simulink model "Missile_Trim_Verification"  (R2021b)
settings: Solver=ode4  StartTime=0.0  StopTime=20  FixedStep=Step_Size  RelTol=1e-3
InitFcn:
  | Missile_Data;
  | Sim_Parameters;
values from neighbouring files (symbols this model uses):
  Init_Euler = x_trim(7:9)    [Sim_Parameters.m]
  Init_Rate = x_trim(4:6)    [Sim_Parameters.m]
  Init_Vel = x_trim(1:3)    [Sim_Parameters.m]
  UNIT_GRAV = 9.81    [Sim_Parameters.m]
undefined symbols (not defined in the file or in its folder): CTC, D, G_turn, gamma_trim, h_trim, Mass, psi_dot_trim, ROC, S, SC, Tbl_CL_ALPHAT, Tbl_CL_DEL_R, Tbl_CL_P, Tbl_CM_0, Tbl_CM_DEL_P, Tbl_CM_PHIT, Tbl_CM_Q, Tbl_CN_DEL_Y, Tbl_CN_PHIT, Tbl_CN_R, Tbl_CX_0, Tbl_CX_ALPHAT, Tbl_CX_DEL_EFF, Tbl_CY_DEL_Y, Tbl_CY_PHIT, Tbl_CZ_0, Tbl_CZ_DEL_P, Tbl_CZ_PHIT, Tbl_SOS, theta_dot_trim, u_trim, V_speed_trim, XCG, XREF
libraries: aerolibasang x3, simulink_extras x3, UAS_Model_library x2, sharedutil x2, shared6dofsys x1, sharedtransform x1
settings Model: Creator=Tiga  LastModifiedBy=Tiga

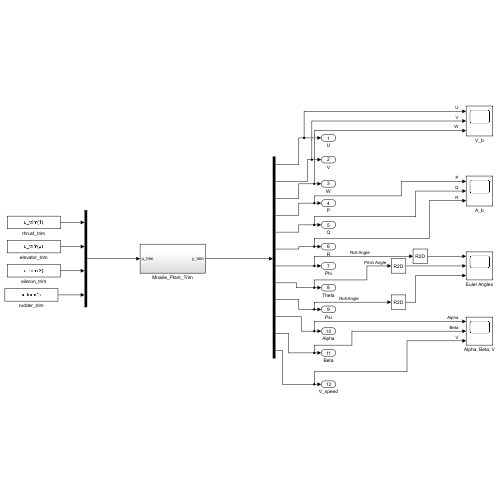
[thumbnail: Simulink's stored preview of the top-level diagram]
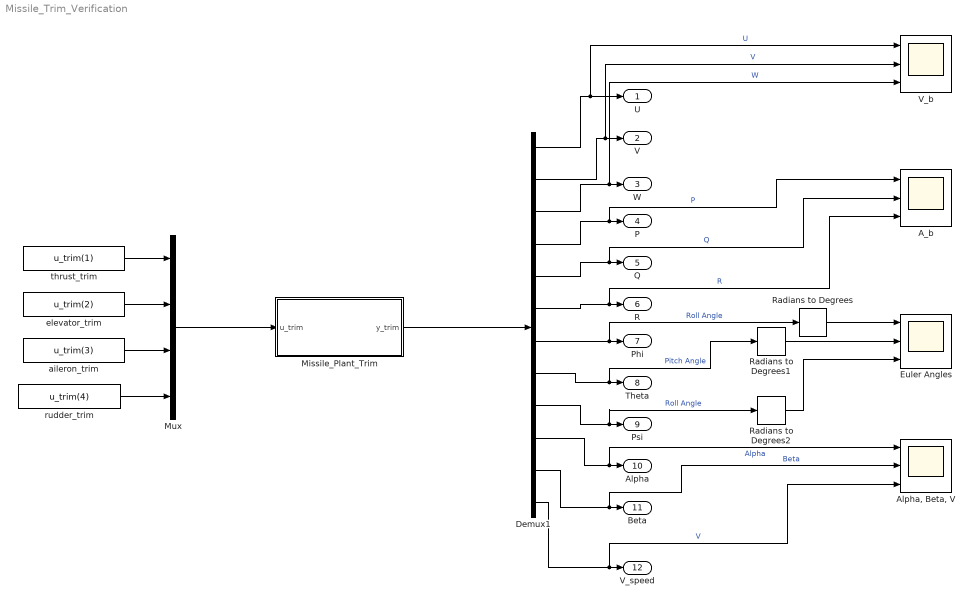
== system Missile_Trim_Verification ==
  A_b : Scope  NumInputPorts=3
  "Alpha, Beta, V" : Scope  NumInputPorts=3
  Demux1 : Demux  Outputs=12
  Euler Angles : Scope  NumInputPorts=3
  Missile_Plant_Trim : Subsystem
  Mux : Mux
  Radians to Degrees : simulink_extras/Transformations/Radians to Degrees
  Radians to Degrees1 : simulink_extras/Transformations/Radians to Degrees
  Radians to Degrees2 : simulink_extras/Transformations/Radians to Degrees
  V_b : Scope  NumInputPorts=3
  aileron_trim : Constant  Value=u_trim(3)
  elevator_trim : Constant  Value=u_trim(2)
  rudder_trim : Constant  Value=u_trim(4)
  thrust_trim : Constant  Value=u_trim(1)
  U : Outport
  V : Outport  Port=2
  W : Outport  Port=3
  P : Outport  Port=4
  Q : Outport  Port=5
  R : Outport  Port=6
  Phi : Outport  Port=7
  Theta : Outport  Port=8
  Psi : Outport  Port=9
  Alpha : Outport  Port=10
  Beta : Outport  Port=11
  V_speed : Outport  Port=12
  wires:
  Mux/1 -> Missile_Plant_Trim/1(u_trim)
  Missile_Plant_Trim/1(y_trim) -> Demux1/1
  Demux1/1 -> U/1, V_b/1  "U"
  Demux1/2 -> V/1, V_b/2  "V"
  Demux1/3 -> W/1, V_b/3  "W"
  Demux1/4 -> A_b/1, P/1  "P"
  Demux1/5 -> A_b/2, Q/1  "Q"
  Demux1/6 -> A_b/3, R/1  "R"
  Demux1/7 -> Radians to Degrees/1, Phi/1  "Roll Angle"
  Demux1/8 -> Radians to Degrees1/1, Theta/1  "Pitch Angle"
  Demux1/9 -> Radians to Degrees2/1, Psi/1  "Roll Angle"
  Demux1/10 -> "Alpha, Beta, V"/1, Alpha/1  "Alpha"
  Demux1/11 -> "Alpha, Beta, V"/2, Beta/1  "Beta"
  Demux1/12 -> "Alpha, Beta, V"/3, V_speed/1  "V"
  thrust_trim/1 -> Mux/1
  elevator_trim/1 -> Mux/2
  aileron_trim/1 -> Mux/3
  rudder_trim/1 -> Mux/4
  Radians to Degrees/1 -> Euler Angles/1
  Radians to Degrees1/1 -> Euler Angles/2
  Radians to Degrees2/1 -> Euler Angles/3

== system Missile_Trim_Verification/Missile_Plant_Trim ==
  u_trim : Inport
  Bus Creator1 : BusCreator  Inputs=3
  Demux2 : Demux
  Environment Model : Subsystem
  Missile Dynamics : Subsystem
  Propulsion Model : Subsystem
  y_trim : Outport
  wires:
  Environment Model/1(speed_of_sound) -> Missile Dynamics/1(speed_of_sound)
  Missile Dynamics/1(y_trim) -> y_trim/1
  u_trim/1 -> Demux2/1
  Environment Model/2(Rho) -> Missile Dynamics/2(Rho)
  Demux2/4 -> Bus Creator1/3  "rudder_trim"
  Bus Creator1/1 -> Missile Dynamics/3(CtrlSurfaces)
  Demux2/1 -> Propulsion Model/1(Desired_Thrust)  "thrust_trim"
  Propulsion Model/1(Propulsion_Thrust) -> Missile Dynamics/4(Propulsion_Thrust)
  Demux2/2 -> Bus Creator1/2  "elevator_trim"
  Demux2/3 -> Bus Creator1/1  "alieron_trim"

== system Missile_Trim_Verification/Missile_Plant_Trim/Environment Model ==
  Atmosphere Model : UAS_Model_library/Envrionment/Atmosphere Model  SystemSampleTime=-1  VariantActivationTime=update diagram  Latency=0  AutoFrameSizeCalculation=off
  Constant : Constant  Value=h_trim
  Interpolation Using Prelookup : Interpolation_n-D  NumberOfTableDimensions=1  Table=Tbl_SOS  InternalRulePriority=Speed
      settings: InputPortMap=u0,u1
  Prelookup : PreLookup  BreakpointsData=Tbl_ALT  ExtrapMethod=Linear
  Terminator : Terminator
  speed_of_sound : Outport  Unit=m/s  VectorParamsAs1DForOutWhenUnconnected=off
  Rho : Outport  Port=2  Unit=kg/m^3  VectorParamsAs1DForOutWhenUnconnected=off
  wires:
  Constant/1 -> Prelookup/1, Atmosphere Model/1
  Prelookup/1 -> Interpolation Using Prelookup/1
  Prelookup/2 -> Interpolation Using Prelookup/2
  Interpolation Using Prelookup/1 -> speed_of_sound/1
  Atmosphere Model/2 -> Rho/1
  Atmosphere Model/1 -> Terminator/1

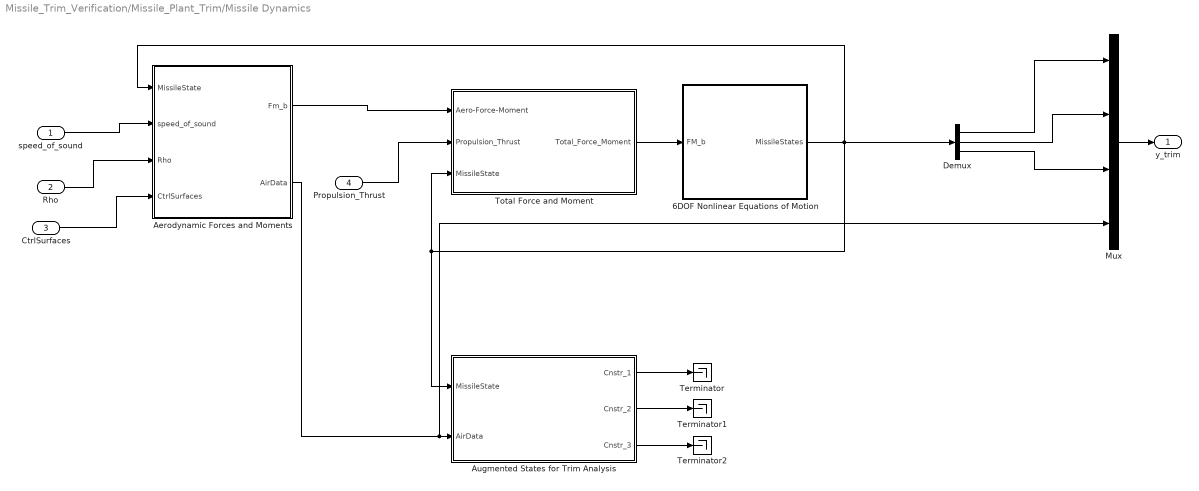
== system Missile_Trim_Verification/Missile_Plant_Trim/Missile Dynamics ==
  speed_of_sound : Inport
  Rho : Inport  Port=2
  CtrlSurfaces : Inport  Port=3
  Propulsion_Thrust : Inport  Port=4
  6DOF Nonlinear Equations of Motion : Subsystem
  Aerodynamic Forces and Moments : Subsystem
  Augmented States for Trim Analysis : Subsystem
  Demux : Demux  Outputs=3
  Mux : Mux
  Terminator : Terminator
  Terminator1 : Terminator
  Terminator2 : Terminator
  Total Force and Moment : Subsystem
  y_trim : Outport
  wires:
  CtrlSurfaces/1 -> Aerodynamic Forces and Moments/4(CtrlSurfaces)
  Rho/1 -> Aerodynamic Forces and Moments/3(Rho)
  speed_of_sound/1 -> Aerodynamic Forces and Moments/2(speed_of_sound)
  Propulsion_Thrust/1 -> Total Force and Moment/2(Propulsion_Thrust)
  Aerodynamic Forces and Moments/1(Fm_b) -> Total Force and Moment/1(Aero-Force-Moment)
  Total Force and Moment/1(Total_Force_Moment) -> 6DOF Nonlinear Equations of Motion/1(FM_b)
  Aerodynamic Forces and Moments/2(AirData) -> Mux/4, Augmented States for Trim Analysis/2(AirData)
  6DOF Nonlinear Equations of Motion/1(MissileStates) -> Demux/1, Augmented States for Trim Analysis/1(MissileState), Total Force and Moment/3(MissileState), Aerodynamic Forces and Moments/1(MissileState)
  Augmented States for Trim Analysis/1(Cnstr_1) -> Terminator/1
  Augmented States for Trim Analysis/2(Cnstr_2) -> Terminator1/1
  Augmented States for Trim Analysis/3(Cnstr_3) -> Terminator2/1
  Demux/1 -> Mux/1
  Demux/2 -> Mux/2
  Demux/3 -> Mux/3
  Mux/1 -> y_trim/1

== system Missile_Trim_Verification/Missile_Plant_Trim/Propulsion Model ==
  note: F_Tx
  Desired_Thrust : Inport
  F_Ty : Constant  Value=0
  F_Tz : Constant  Value=0
  L_T : Constant  Value=0
  M_T : Constant  Value=0
  Mux : Mux  Inputs=3
  Mux1 : Mux  Inputs=3
  Mux2 : Mux  Inputs=2
  N_T : Constant  Value=0
  Propulsion_Thrust : Outport
  wires:
  N_T/1 -> Mux1/3
  M_T/1 -> Mux1/2
  L_T/1 -> Mux1/1
  F_Tz/1 -> Mux/3
  F_Ty/1 -> Mux/2
  Desired_Thrust/1 -> Mux/1
  Mux2/1 -> Propulsion_Thrust/1
  Mux1/1 -> Mux2/2
  Mux/1 -> Mux2/1

== system Missile_Trim_Verification/Missile_Plant_Trim/Missile Dynamics/6DOF Nonlinear Equations of Motion ==
  FM_b : Inport
  Calculate Euler Angles : Subsystem  AncestorBlock=UAS_Model_library/Equations of Motion/Calculate DCM & Euler Angles
  Calculate omega_dot : shared6dofsys/Calculate omega_dot  aMode=aMode
      settings: SourceProductBaseCode=AE
  Demux2 : Demux  Outputs=2
  "Determine Force, Moment & Inertia" : UAS_Model_library/Equations of Motion/Determine Force, Moment & Inertia  SystemSampleTime=-1  VariantActivationTime=update diagram  Latency=0  AutoFrameSizeCalculation=off
  Mux : Mux  Inputs=3
  Product : Product  Inputs=*/  SaturateOnIntegerOverflow=on  OutDataTypeStr=Inherit: Same as first input
  Sum : Sum  Inputs=|++  SaturateOnIntegerOverflow=on
  Vbxw : sharedutil/3x3 Cross Product  aMode=aMode
      settings: SourceProductBaseCode=AE,PW,DR,MT,UV,VE
  "p,q,r " : Integrator  InitialCondition=Init_Rate
  ub,vb,wb : Integrator  InitialCondition=Init_Vel
  MissileStates : Outport
  wires:
  Demux2/2 -> Calculate omega_dot/3  "M_b"
  FM_b/1 -> Demux2/1
  Demux2/1 -> "Determine Force, Moment & Inertia"/1  "F_b"
  "Determine Force, Moment & Inertia"/1 -> Product/1
  "Determine Force, Moment & Inertia"/2 -> Product/2
  "Determine Force, Moment & Inertia"/3 -> Calculate omega_dot/2
  Sum/1 -> ub,vb,wb/1
  "p,q,r "/1 -> Vbxw/2, Mux/2, Calculate omega_dot/1, Calculate Euler Angles/1("p q r ")  "A_b"
  ub,vb,wb/1 -> Mux/1, Vbxw/1  "V_b"
  Calculate omega_dot/1 -> "p,q,r "/1
  Vbxw/1 -> Sum/2
  Product/1 -> Sum/1
  Calculate Euler Angles/1(Euler) -> Mux/3  "Euler_angles"
  Mux/1 -> MissileStates/1

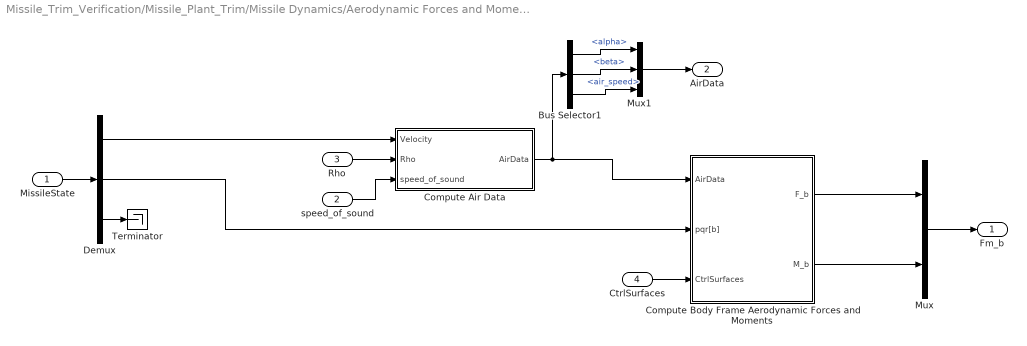
== system Missile_Trim_Verification/Missile_Plant_Trim/Missile Dynamics/Aerodynamic Forces and Moments ==
  MissileState : Inport
  speed_of_sound : Inport  Port=2  Unit=m/s
  Rho : Inport  Port=3  Unit=kg/m^3
  CtrlSurfaces : Inport  Port=4
  Bus Selector1 : BusSelector  OutputSignals=alpha,beta,air_speed
  Compute Air Data : Subsystem
  Compute Body Frame Aerodynamic Forces and Moments : Subsystem
  Demux : Demux  Outputs=3
  Mux : Mux  Inputs=2
  Mux1 : Mux  Inputs=3
  Terminator : Terminator
  Fm_b : Outport
  AirData : Outport  Port=2
  wires:
  Compute Body Frame Aerodynamic Forces and Moments/1(F_b) -> Mux/1
  Compute Body Frame Aerodynamic Forces and Moments/2(M_b) -> Mux/2
  Mux/1 -> Fm_b/1
  CtrlSurfaces/1 -> Compute Body Frame Aerodynamic Forces and Moments/3(CtrlSurfaces)
  Compute Air Data/1(AirData) -> Bus Selector1/1, Compute Body Frame Aerodynamic Forces and Moments/1(AirData)
  speed_of_sound/1 -> Compute Air Data/3(speed_of_sound)
  Rho/1 -> Compute Air Data/2(Rho)
  Demux/1 -> Compute Air Data/1(Velocity)
  Bus Selector1/2 -> Mux1/2  "<beta>"
  Mux1/1 -> AirData/1
  MissileState/1 -> Demux/1
  Demux/3 -> Terminator/1
  Demux/2 -> Compute Body Frame Aerodynamic Forces and Moments/2(pqr[b])
  Bus Selector1/1 -> Mux1/1  "<alpha>"
  Bus Selector1/3 -> Mux1/3  "<air_speed>"

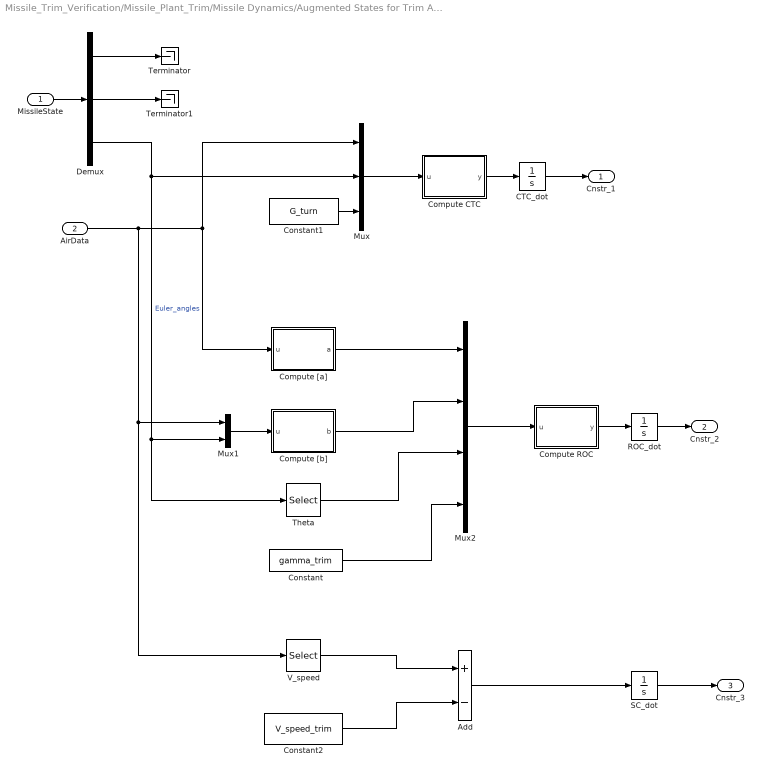
== system Missile_Trim_Verification/Missile_Plant_Trim/Missile Dynamics/Augmented States for Trim Analysis ==
  MissileState : Inport
  AirData : Inport  Port=2
  Add : Sum  Inputs=+-
  CTC_dot : Integrator  InitialCondition=CTC
  Compute CTC : MATLAB Function  TreatAsAtomicUnit=on
  Compute ROC : MATLAB Function  TreatAsAtomicUnit=on
  Compute [a] : MATLAB Function  TreatAsAtomicUnit=on
  Compute [b] : MATLAB Function  TreatAsAtomicUnit=on
  Constant : Constant  Value=gamma_trim
  Constant1 : Constant  Value=G_turn
  Constant2 : Constant  Value=V_speed_trim
  Demux : Demux  Outputs=3
  Mux : Mux  Inputs=3
  Mux1 : Mux  Inputs=2
  Mux2 : Mux
  ROC_dot : Integrator  InitialCondition=ROC
  SC_dot : Integrator  InitialCondition=SC
  Terminator : Terminator
  Terminator1 : Terminator
  Theta : Selector  InputPortWidth=3  IndexOptions=Index vector (dialog)  Indices=[2]  OutputSizes=1
  V_speed : Selector  InputPortWidth=3  IndexOptions=Index vector (dialog)  Indices=[3]  OutputSizes=1
  Cnstr_1 : Outport
  Cnstr_2 : Outport  Port=2
  Cnstr_3 : Outport  Port=3
  wires:
  MissileState/1 -> Demux/1
  Demux/1 -> Terminator/1
  Demux/2 -> Terminator1/1
  AirData/1 -> Mux1/1, V_speed/1, Compute [a]/1(u), Mux/1
  Demux/3 -> Mux/2, Theta/1, Mux1/2  "Euler_angles"
  Constant1/1 -> Mux/3
  Mux/1 -> Compute CTC/1(u)
  Compute CTC/1(y) -> CTC_dot/1
  CTC_dot/1 -> Cnstr_1/1
  Mux1/1 -> Compute [b]/1(u)
  Compute [a]/1(a) -> Mux2/1
  Compute [b]/1(b) -> Mux2/2
  Theta/1 -> Mux2/3
  Constant/1 -> Mux2/4
  Mux2/1 -> Compute ROC/1(u)
  Compute ROC/1(y) -> ROC_dot/1
  ROC_dot/1 -> Cnstr_2/1
  V_speed/1 -> Add/1
  Constant2/1 -> Add/2
  Add/1 -> SC_dot/1
  SC_dot/1 -> Cnstr_3/1

== system Missile_Trim_Verification/Missile_Plant_Trim/Missile Dynamics/Total Force and Moment ==
  Aero-Force-Moment : Inport
  Propulsion_Thrust : Inport  Port=2
  MissileState : Inport  Port=3
  Demux : Demux  Outputs=2
  Demux1 : Demux  Outputs=2
  Gravity : Subsystem
  Gravity's effect on moment : Constant  Value=0
  Mux : Mux  Inputs=2
  Total Force : Sum  Inputs=+++
  Total Moment : Sum  Inputs=+++
  Total_Force_Moment : Outport
  wires:
  Aero-Force-Moment/1 -> Demux/1
  Propulsion_Thrust/1 -> Demux1/1
  Demux/1 -> Total Force/1  "Aero-F"
  Demux1/1 -> Total Force/2  "Prop-F"
  MissileState/1 -> Gravity/1(MissileState)
  Gravity/1(Gravitational Force) -> Total Force/3  "Gravity-F"
  Demux/2 -> Total Moment/1  "Aero-M"
  Demux1/2 -> Total Moment/2  "Prop-M"
  Gravity's effect on moment/1 -> Total Moment/3
  Total Force/1 -> Mux/1
  Total Moment/1 -> Mux/2
  Mux/1 -> Total_Force_Moment/1

== system Missile_Trim_Verification/Missile_Plant_Trim/Missile Dynamics/6DOF Nonlinear Equations of Motion/Calculate Euler Angles ==
  "p q r " : Inport
  Demux : Demux  Outputs=3
  Mux : Mux  Inputs=3
  Pull-up Constraint : Constant  Value=theta_dot_trim
  Subsystem : Subsystem
  Sum : Sum  Inputs=|++
  Sum1 : Sum  Inputs=|++
  Turn rate Constraint : Constant  Value=psi_dot_trim
  phi theta psi : Integrator  InitialCondition=Init_Euler
  Euler : Outport  VectorParamsAs1DForOutWhenUnconnected=off
  wires:
  phi theta psi/1 -> Subsystem/2(phi theta psi1), Euler/1
  "p q r "/1 -> Subsystem/1(p q r)
  Subsystem/1(phidot thetadot psi) -> Demux/1
  Demux/1 -> Mux/1
  Pull-up Constraint/1 -> Sum/2
  Demux/2 -> Sum/1
  Sum/1 -> Mux/2
  Turn rate Constraint/1 -> Sum1/2
  Demux/3 -> Sum1/1
  Sum1/1 -> Mux/3
  Mux/1 -> phi theta psi/1

== system Missile_Trim_Verification/Missile_Plant_Trim/Missile Dynamics/Aerodynamic Forces and Moments/Compute Air Data ==
  Velocity : Inport
  Rho : Inport  Port=2  Unit=kg/m^3
  speed_of_sound : Inport  Port=3  Unit=m/s
  Bus Creator : BusCreator  Inputs=5
  Dynamic Pressure : aerolibasang/Dynamic Pressure
  "Incidence, Sideslip, & Airspeed" : aerolibasang/Incidence, Sideslip, & Airspeed
  Mach Number : aerolibasang/Mach Number
      settings: SourceProductBaseCode=AE
  AirData : Outport
  wires:
  "Incidence, Sideslip, & Airspeed"/3 -> Bus Creator/3  "air_speed"
  Bus Creator/1 -> AirData/1
  speed_of_sound/1 -> Mach Number/2
  "Incidence, Sideslip, & Airspeed"/2 -> Bus Creator/2  "beta"
  Dynamic Pressure/1 -> Bus Creator/4  "dynamic_pressure"
  "Incidence, Sideslip, & Airspeed"/1 -> Bus Creator/1  "alpha"
  Rho/1 -> Dynamic Pressure/2
  Mach Number/1 -> Bus Creator/5  "mach"
  Velocity/1 -> Dynamic Pressure/1, Mach Number/1, "Incidence, Sideslip, & Airspeed"/1

== system Missile_Trim_Verification/Missile_Plant_Trim/Missile Dynamics/Aerodynamic Forces and Moments/Compute Body Frame Aerodynamic Forces and Moments ==
  AirData : Inport
  pqr[b] : Inport  Port=2
  CtrlSurfaces : Inport  Port=3
  Bus Selector : BusSelector  OutputSignals=dynamic_pressure
  Compute Aeroballistics Frame Aerodynamics Coefficients : Subsystem
  Compute Body Frame Aerodynamic Forces and Moments : Subsystem
  Convert AeroCoeffs_a to AeroCoeffs_b : Subsystem
  Display : Display
  F_b : Outport
  M_b : Outport  Port=2
  wires:
  Convert AeroCoeffs_a to AeroCoeffs_b/2(Aero-M-Coeffs_b) -> Compute Body Frame Aerodynamic Forces and Moments/3(Aero-M-Coeffs_b)
  Compute Aeroballistics Frame Aerodynamics Coefficients/2(Aero-M-Coeffs_a) -> Convert AeroCoeffs_a to AeroCoeffs_b/2(Aero-M-Coeffs_a)
  Compute Aeroballistics Frame Aerodynamics Coefficients/3(ROT_b_to_a) -> Convert AeroCoeffs_a to AeroCoeffs_b/3(ROT_b_to_a)
  Bus Selector/1 -> Compute Body Frame Aerodynamic Forces and Moments/1(dynamic_pressure)  "<dynamic_pressure>"
  Compute Body Frame Aerodynamic Forces and Moments/2(M_b) -> M_b/1
  Convert AeroCoeffs_a to AeroCoeffs_b/1(Aero-F-Coeffs_b) -> Compute Body Frame Aerodynamic Forces and Moments/2(Aero-F-Coeffs_b)
  Compute Body Frame Aerodynamic Forces and Moments/1(F_b) -> F_b/1
  Compute Aeroballistics Frame Aerodynamics Coefficients/1(Aero-F-Coeffs_a) -> Convert AeroCoeffs_a to AeroCoeffs_b/1(Aero-F-Coeffs_a)
  pqr[b]/1 -> Compute Aeroballistics Frame Aerodynamics Coefficients/2(pqr[b])
  CtrlSurfaces/1 -> Compute Aeroballistics Frame Aerodynamics Coefficients/3(CtrlSurfaces)
  AirData/1 -> Display/1, Compute Aeroballistics Frame Aerodynamics Coefficients/1(AirData), Bus Selector/1

== system Missile_Trim_Verification/Missile_Plant_Trim/Missile Dynamics/Total Force and Moment/Gravity ==
  MissileState : Inport
  Constant : Constant  Value=Mass
  Constant1 : Constant  Value=0
  Demux : Demux  Outputs=3
  EulerAngle to ROT_e_to_b : Subsystem
  Matrix Multiply : Product  Multiplication=Matrix(*)
  Mux : Mux  Inputs=3
  Terminator : Terminator
  Terminator1 : Terminator
  UNIT_GRAV : Gain  Gain=UNIT_GRAV
  Gravitational Force : Outport
  wires:
  UNIT_GRAV/1 -> Mux/3
  Constant/1 -> UNIT_GRAV/1
  Constant1/1 -> Mux/2, Mux/1
  Mux/1 -> Matrix Multiply/2
  Matrix Multiply/1 -> Gravitational Force/1
  EulerAngle to ROT_e_to_b/1(DCM_be) -> Matrix Multiply/1
  MissileState/1 -> Demux/1
  Demux/1 -> Terminator/1
  Demux/2 -> Terminator1/1
  Demux/3 -> EulerAngle to ROT_e_to_b/1(Euler)

== system Missile_Trim_Verification/Missile_Plant_Trim/Missile Dynamics/6DOF Nonlinear Equations of Motion/Calculate Euler Angles/Subsystem ==
  p q r : Inport
  phi theta psi1 : Inport  Port=2
  Mux1 : Mux  Inputs=[3 3 3]
  Mux2 : Mux  Inputs=3
  phidot : Fcn  Expr=u[1]+(u[2]*u[4]+u[3]*u[7])*(u[5]/u[8])
  psidot : Fcn  Expr=(u[2]*u[4]+u[3]*u[7])/u[8]
  sincos : Trigonometry  Operator=sincos
  thetadot : Fcn  Expr=u[2]*u[7]-u[3]*u[4]
  phidot thetadot psi : Outport  InitialOutput=0  VectorParamsAs1DForOutWhenUnconnected=off
  wires:
  phi theta psi1/1 -> sincos/1
  psidot/1 -> Mux2/3
  sincos/2 -> Mux1/3
  Mux1/1 -> psidot/1, phidot/1, thetadot/1
  thetadot/1 -> Mux2/2
  phidot/1 -> Mux2/1
  Mux2/1 -> phidot thetadot psi/1
  sincos/1 -> Mux1/2
  p q r/1 -> Mux1/1

== system Missile_Trim_Verification/Missile_Plant_Trim/Missile Dynamics/Aerodynamic Forces and Moments/Compute Body Frame Aerodynamic Forces and Moments/Compute Aeroballistics Frame Aerodynamics Coefficients ==
  AirData : Inport
  pqr[b] : Inport  Port=2
  CtrlSurfaces : Inport  Port=3
  Calculate Coefficient Parameters : Subsystem
  Compute Aero-F-Coeffs_a : Subsystem
  Compute Aero-M-Coeffs_a : Subsystem
  Mach_Number Index Search : PreLookup  BreakpointsData=Tbl_MACH  OutputSelection=Index and fraction as bus  ExtrapMethod=Linear
  alpha_T Index Search : PreLookup  BreakpointsData=Tbl_ALPHAT  OutputSelection=Index and fraction as bus  BeginIndexSearchUsingPreviousIndexResult=on  ExtrapMethod=Linear
  Aero-F-Coeffs_a : Outport
  Aero-M-Coeffs_a : Outport  Port=2
  ROT_b_to_a : Outport  Port=3
  wires:
  Compute Aero-M-Coeffs_a/1(Aero-M-Coeffs_a) -> Aero-M-Coeffs_a/1
  Calculate Coefficient Parameters/9(pqr[a]) -> Compute Aero-M-Coeffs_a/8(pqr[a])
  Calculate Coefficient Parameters/8(geo_param) -> Compute Aero-M-Coeffs_a/7(geo_param)
  Calculate Coefficient Parameters/7(D/2V) -> Compute Aero-M-Coeffs_a/6(D/2V)
  Compute Aero-F-Coeffs_a/1(Aero-F-Coeffs_a) -> Aero-F-Coeffs_a/1, Compute Aero-M-Coeffs_a/9(Aero-F-Coeffs_a)
  Calculate Coefficient Parameters/6(roll_angle_T) -> Compute Aero-M-Coeffs_a/3(roll_angle_T), Compute Aero-F-Coeffs_a/4(roll_angle_T)
  Calculate Coefficient Parameters/5(CtrlSurfaces[a]) -> Compute Aero-M-Coeffs_a/5(CtrlSurfaces[a]), Compute Aero-F-Coeffs_a/6(CtrlSurfaces[a])
  Calculate Coefficient Parameters/4(dEFF) -> Compute Aero-F-Coeffs_a/5(dEFF)
  Mach_Number Index Search/1 -> Compute Aero-F-Coeffs_a/2(Mach_Number_index), Compute Aero-M-Coeffs_a/2(Mach_Number_index)
  alpha_T Index Search/1 -> Compute Aero-F-Coeffs_a/1(alpha_T_index), Compute Aero-M-Coeffs_a/1(alpha_T_index)
  Calculate Coefficient Parameters/3(Mach_Number) -> Mach_Number Index Search/1
  Calculate Coefficient Parameters/2(alpha_T) -> Compute Aero-F-Coeffs_a/3(alpha_T), Compute Aero-M-Coeffs_a/4(alpha_T), alpha_T Index Search/1
  Calculate Coefficient Parameters/1(ROT_b_to_a) -> ROT_b_to_a/1
  AirData/1 -> Calculate Coefficient Parameters/1(AirData)
  pqr[b]/1 -> Calculate Coefficient Parameters/2(pqr[b])
  CtrlSurfaces/1 -> Calculate Coefficient Parameters/3(CtrlSurfaces[b])

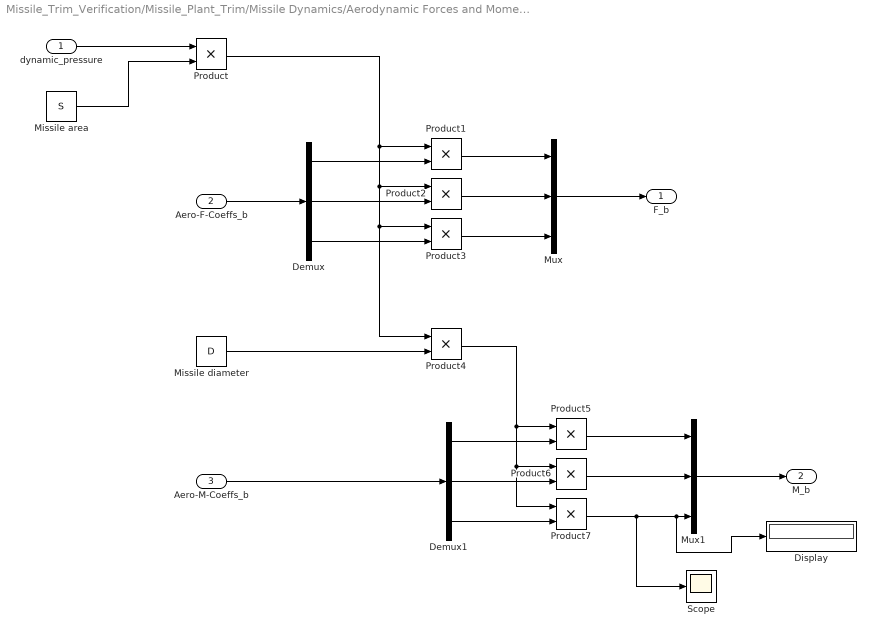
== system Missile_Trim_Verification/Missile_Plant_Trim/Missile Dynamics/Aerodynamic Forces and Moments/Compute Body Frame Aerodynamic Forces and Moments/Compute Body Frame Aerodynamic Forces and Moments ==
  dynamic_pressure : Inport
  Aero-F-Coeffs_b : Inport  Port=2
  Aero-M-Coeffs_b : Inport  Port=3
  Demux : Demux  Outputs=3
  Demux1 : Demux  Outputs=3
  Display : Display
  Missile area : Constant  Value=S
  "Missile diameter " : Constant  Value=D
  Mux : Mux  Inputs=3
  Mux1 : Mux  Inputs=3
  Product{,1..7} (8 alike) : Product
  Scope : Scope
  F_b : Outport
  M_b : Outport  Port=2
  wires:
  Product7/1 -> Scope/1, Display/1, Mux1/3
  Demux1/3 -> Product7/2
  Product6/1 -> Mux1/2
  Demux1/2 -> Product6/2
  Product5/1 -> Mux1/1
  Demux1/1 -> Product5/2
  Product4/1 -> Product5/1, Product7/1, Product6/1
  "Missile diameter "/1 -> Product4/2
  Mux1/1 -> M_b/1
  Product3/1 -> Mux/3
  Demux/3 -> Product3/2
  Product2/1 -> Mux/2
  Demux/2 -> Product2/2
  Product1/1 -> Mux/1
  Demux/1 -> Product1/2
  Product/1 -> Product1/1, Product2/1, Product3/1, Product4/1
  Missile area/1 -> Product/2
  dynamic_pressure/1 -> Product/1
  Mux/1 -> F_b/1
  Aero-M-Coeffs_b/1 -> Demux1/1
  Aero-F-Coeffs_b/1 -> Demux/1

== system Missile_Trim_Verification/Missile_Plant_Trim/Missile Dynamics/Aerodynamic Forces and Moments/Compute Body Frame Aerodynamic Forces and Moments/Convert AeroCoeffs_a to AeroCoeffs_b ==
  Aero-F-Coeffs_a : Inport
  Aero-M-Coeffs_a : Inport  Port=2
  ROT_b_to_a : Inport  Port=3
  Bus to Vector : BusToVector
  Bus to Vector1 : BusToVector
  Matrix Multiply : Product  Multiplication=Matrix(*)
  Matrix Multiply1 : Product  Multiplication=Matrix(*)
  ROT_a_to_b : Math  Operator=transpose  SaturateOnIntegerOverflow=on
  Reshape : Reshape  OutputDimensionality=Column vector (2-D)
  Reshape1 : Reshape  OutputDimensionality=Column vector (2-D)
  Aero-F-Coeffs_b : Outport
  Aero-M-Coeffs_b : Outport  Port=2
  wires:
  Bus to Vector1/1 -> Reshape1/1
  Aero-M-Coeffs_a/1 -> Bus to Vector1/1
  Bus to Vector/1 -> Reshape/1
  Aero-F-Coeffs_a/1 -> Bus to Vector/1
  Reshape1/1 -> Matrix Multiply1/2
  Reshape/1 -> Matrix Multiply/2
  ROT_a_to_b/1 -> Matrix Multiply1/1, Matrix Multiply/1
  Matrix Multiply1/1 -> Aero-M-Coeffs_b/1
  Matrix Multiply/1 -> Aero-F-Coeffs_b/1
  ROT_b_to_a/1 -> ROT_a_to_b/1

== system Missile_Trim_Verification/Missile_Plant_Trim/Missile Dynamics/Total Force and Moment/Gravity/EulerAngle to ROT_e_to_b ==
  Euler : Inport
  Rotation Angles to Direction Cosine Matrix : sharedtransform/Rotation Angles to Direction Cosine Matrix  rotationOrder=ZYX  aMode=aMode
      settings: SourceProductBaseCode=AE,PW,DR,MT,UV,VE
  Selector : Selector  InputPortWidth=3  IndexOptions=Index vector (dialog)  Indices=[3 2 1]  OutputSizes=1
  DCM_be : Outport
  wires:
  Euler/1 -> Selector/1
  Selector/1 -> Rotation Angles to Direction Cosine Matrix/1  "3 (rad)"
  Rotation Angles to Direction Cosine Matrix/1 -> DCM_be/1

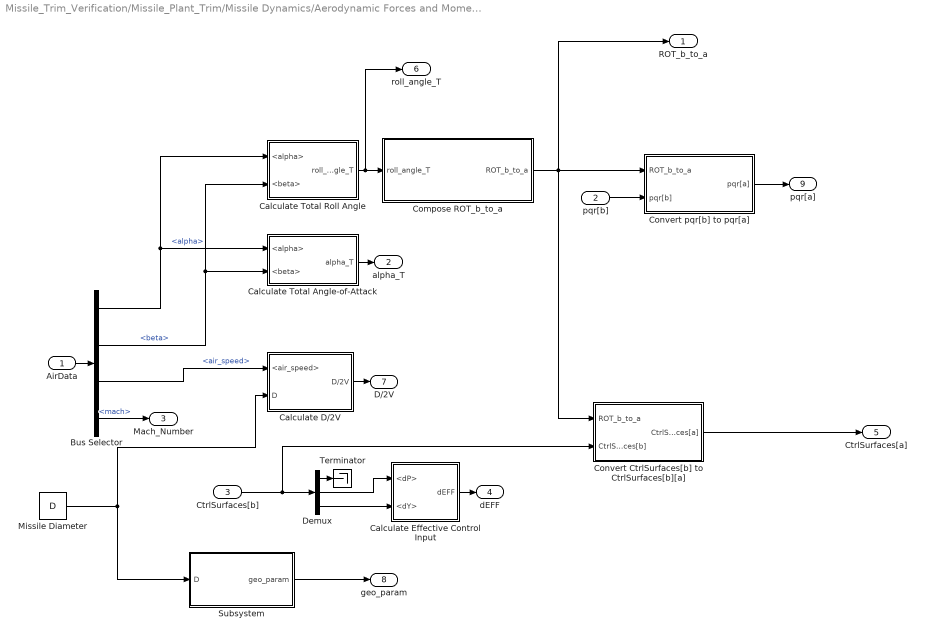
== system Missile_Trim_Verification/Missile_Plant_Trim/Missile Dynamics/Aerodynamic Forces and Moments/Compute Body Frame Aerodynamic Forces and Moments/Compute Aeroballistics Frame Aerodynamics Coefficients/Calculate Coefficient Parameters ==
  AirData : Inport
  pqr[b] : Inport  Port=2
  CtrlSurfaces[b] : Inport  Port=3
  Bus Selector : BusSelector  OutputSignals=alpha,beta,air_speed,mach
  Calculate D/2V : Subsystem
  Calculate Effective Control Input : Subsystem
  Calculate Total Angle-of-Attack : Subsystem
  Calculate Total Roll Angle : Subsystem
  Compose ROT_b_to_a : Subsystem
  Convert CtrlSurfaces[b] to CtrlSurfaces[b][a] : Subsystem
  Convert pqr[b] to pqr[a] : Subsystem
  Demux : Demux  Outputs=3
  Missile Diameter : Constant  Value=D
  Subsystem : Subsystem
  Terminator : Terminator
  ROT_b_to_a : Outport
  alpha_T : Outport  Port=2
  Mach_Number : Outport  Port=3
  dEFF : Outport  Port=4
  CtrlSurfaces[a] : Outport  Port=5
  roll_angle_T : Outport  Port=6
  D/2V : Outport  Port=7
  geo_param : Outport  Port=8
  pqr[a] : Outport  Port=9
  wires:
  Subsystem/1(geo_param) -> geo_param/1
  Missile Diameter/1 -> Calculate D/2V/2(D), Subsystem/1(D)
  Bus Selector/4 -> Mach_Number/1  "<mach>"
  Bus Selector/3 -> Calculate D/2V/1(<air_speed>)  "<air_speed>"
  Bus Selector/2 -> Calculate Total Angle-of-Attack/2(<beta>), Calculate Total Roll Angle/2(<beta>)  "<beta>"
  Bus Selector/1 -> Calculate Total Angle-of-Attack/1(<alpha>), Calculate Total Roll Angle/1(<alpha>)  "<alpha>"
  AirData/1 -> Bus Selector/1
  Convert CtrlSurfaces[b] to CtrlSurfaces[b][a]/1(CtrlSurfaces[a]) -> CtrlSurfaces[a]/1
  Convert pqr[b] to pqr[a]/1(pqr[a]) -> pqr[a]/1
  Calculate Total Angle-of-Attack/1(alpha_T) -> alpha_T/1
  Calculate Effective Control Input/1(dEFF) -> dEFF/1
  CtrlSurfaces[b]/1 -> Convert CtrlSurfaces[b] to CtrlSurfaces[b][a]/2(CtrlSurfaces[b]), Demux/1
  Calculate Total Roll Angle/1(roll_angle_T) -> roll_angle_T/1, Compose ROT_b_to_a/1(roll_angle_T)
  Calculate D/2V/1(D/2V) -> D/2V/1
  pqr[b]/1 -> Convert pqr[b] to pqr[a]/2(pqr[b])
  Compose ROT_b_to_a/1(ROT_b_to_a) -> Convert pqr[b] to pqr[a]/1(ROT_b_to_a), Convert CtrlSurfaces[b] to CtrlSurfaces[b][a]/1(ROT_b_to_a), ROT_b_to_a/1
  Demux/1 -> Terminator/1
  Demux/2 -> Calculate Effective Control Input/1(<dP>)
  Demux/3 -> Calculate Effective Control Input/2(<dY>)

== system Missile_Trim_Verification/Missile_Plant_Trim/Missile Dynamics/Aerodynamic Forces and Moments/Compute Body Frame Aerodynamic Forces and Moments/Compute Aeroballistics Frame Aerodynamics Coefficients/Compute Aero-F-Coeffs_a ==
  alpha_T_index : Inport
  Mach_Number_index : Inport  Port=2
  alpha_T : Inport  Port=3
  roll_angle_T : Inport  Port=4
  dEFF : Inport  Port=5
  CtrlSurfaces[a] : Inport  Port=6
  Bus Creator : BusCreator  Inputs=3
  Compute CX_a : Subsystem
  Compute CY_a : Subsystem
  Compute CZ_a : Subsystem
  Aero-F-Coeffs_a : Outport
  wires:
  Bus Creator/1 -> Aero-F-Coeffs_a/1
  Compute CZ_a/1(CZ_a) -> Bus Creator/3  "CZ_a"
  Compute CY_a/1(CY_a) -> Bus Creator/2  "CY_a"
  Compute CX_a/1(CX_a) -> Bus Creator/1  "CX_a"
  CtrlSurfaces[a]/1 -> Compute CZ_a/4(CtrlSurfaces[a]), Compute CY_a/4(CtrlSurfaces[a])
  roll_angle_T/1 -> Compute CY_a/3(roll_angle_T), Compute CZ_a/3(roll_angle_T)
  alpha_T_index/1 -> Compute CY_a/1(alpha_T_index), Compute CZ_a/1(alpha_T_index)
  dEFF/1 -> Compute CX_a/3(dEFF)
  alpha_T/1 -> Compute CX_a/2(alpha_T)
  Mach_Number_index/1 -> Compute CX_a/1(Mach_Number_index), Compute CY_a/2(Mach_Number_index), Compute CZ_a/2(Mach_Number_index)

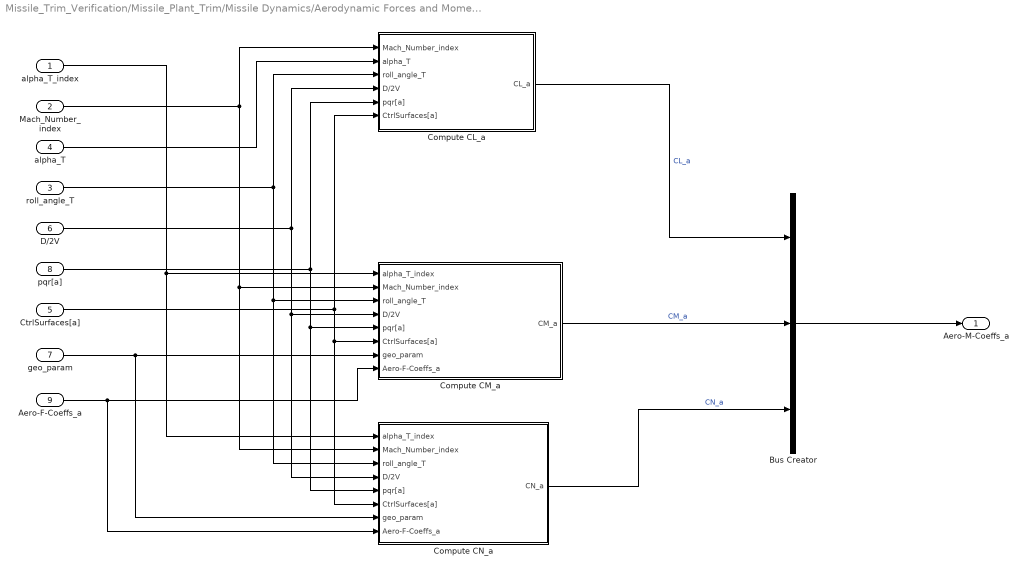
== system Missile_Trim_Verification/Missile_Plant_Trim/Missile Dynamics/Aerodynamic Forces and Moments/Compute Body Frame Aerodynamic Forces and Moments/Compute Aeroballistics Frame Aerodynamics Coefficients/Compute Aero-M-Coeffs_a ==
  alpha_T_index : Inport
  Mach_Number_index : Inport  Port=2
  roll_angle_T : Inport  Port=3
  alpha_T : Inport  Port=4
  CtrlSurfaces[a] : Inport  Port=5
  D/2V : Inport  Port=6
  geo_param : Inport  Port=7
  pqr[a] : Inport  Port=8
  Aero-F-Coeffs_a : Inport  Port=9
  Bus Creator : BusCreator  Inputs=3
  Compute CL_a : Subsystem
  Compute CM_a : Subsystem
  Compute CN_a : Subsystem
  Aero-M-Coeffs_a : Outport
  wires:
  Compute CN_a/1(CN_a) -> Bus Creator/3  "CN_a"
  Compute CM_a/1(CM_a) -> Bus Creator/2  "CM_a"
  Aero-F-Coeffs_a/1 -> Compute CN_a/8(Aero-F-Coeffs_a), Compute CM_a/8(Aero-F-Coeffs_a)
  alpha_T_index/1 -> Compute CN_a/1(alpha_T_index), Compute CM_a/1(alpha_T_index)
  geo_param/1 -> Compute CN_a/7(geo_param), Compute CM_a/7(geo_param)
  Compute CL_a/1(CL_a) -> Bus Creator/1  "CL_a"
  CtrlSurfaces[a]/1 -> Compute CL_a/6(CtrlSurfaces[a]), Compute CN_a/6(CtrlSurfaces[a]), Compute CM_a/6(CtrlSurfaces[a])
  pqr[a]/1 -> Compute CL_a/5(pqr[a]), Compute CN_a/5(pqr[a]), Compute CM_a/5(pqr[a])
  D/2V/1 -> Compute CL_a/4(D/2V), Compute CN_a/4(D/2V), Compute CM_a/4(D/2V)
  roll_angle_T/1 -> Compute CL_a/3(roll_angle_T), Compute CN_a/3(roll_angle_T), Compute CM_a/3(roll_angle_T)
  alpha_T/1 -> Compute CL_a/2(alpha_T)
  Mach_Number_index/1 -> Compute CL_a/1(Mach_Number_index), Compute CN_a/2(Mach_Number_index), Compute CM_a/2(Mach_Number_index)
  Bus Creator/1 -> Aero-M-Coeffs_a/1

== system Missile_Trim_Verification/Missile_Plant_Trim/Missile Dynamics/Aerodynamic Forces and Moments/Compute Body Frame Aerodynamic Forces and Moments/Compute Aeroballistics Frame Aerodynamics Coefficients/Calculate Coefficient Parameters/Calculate D//2V ==
  <air_speed> : Inport
  D : Inport  Port=2
  Divide : Product  Inputs=*/
  Gain : Gain  Gain=2
  D/2V : Outport
  wires:
  D/1 -> Divide/1
  <air_speed>/1 -> Gain/1
  Divide/1 -> D/2V/1
  Gain/1 -> Divide/2

== system Missile_Trim_Verification/Missile_Plant_Trim/Missile Dynamics/Aerodynamic Forces and Moments/Compute Body Frame Aerodynamic Forces and Moments/Compute Aeroballistics Frame Aerodynamics Coefficients/Calculate Coefficient Parameters/Calculate Effective Control Input ==
  <dP> : Inport
  <dY> : Inport  Port=2
  Abs : Abs
  Abs1 : Abs
  Constant : Constant  Value=2
  Divide : Product  Inputs=*/
  Plus : Sum
  dEFF : Outport
  wires:
  <dY>/1 -> Abs1/1
  <dP>/1 -> Abs/1
  Divide/1 -> dEFF/1
  Plus/1 -> Divide/1
  Abs/1 -> Plus/1
  Abs1/1 -> Plus/2
  Constant/1 -> Divide/2

== system Missile_Trim_Verification/Missile_Plant_Trim/Missile Dynamics/Aerodynamic Forces and Moments/Compute Body Frame Aerodynamic Forces and Moments/Compute Aeroballistics Frame Aerodynamics Coefficients/Calculate Coefficient Parameters/Calculate Total Angle-of-Attack ==
  <alpha> : Inport
  <beta> : Inport  Port=2
  Acos : Trigonometry  Operator=acos
  Cos : Trigonometry  Operator=cos
  Cos1 : Trigonometry  Operator=cos
  Display : Display
  Product : Product
  alpha_T : Outport
  wires:
  <alpha>/1 -> Cos/1
  Cos1/1 -> Product/2
  Product/1 -> Acos/1
  Acos/1 -> Display/1, alpha_T/1
  Cos/1 -> Product/1
  <beta>/1 -> Cos1/1

== system Missile_Trim_Verification/Missile_Plant_Trim/Missile Dynamics/Aerodynamic Forces and Moments/Compute Body Frame Aerodynamic Forces and Moments/Compute Aeroballistics Frame Aerodynamics Coefficients/Calculate Coefficient Parameters/Calculate Total Roll Angle ==
  <alpha> : Inport
  <beta> : Inport  Port=2
  Atan2 : Trigonometry  Operator=atan2
  Sin : Trigonometry
  Tan : Trigonometry  Operator=tan
  roll_angle_T : Outport
  wires:
  Atan2/1 -> roll_angle_T/1
  <alpha>/1 -> Sin/1
  Sin/1 -> Atan2/2  "sin(alpha)"
  <beta>/1 -> Tan/1
  Tan/1 -> Atan2/1  "tan(beta)"

== system Missile_Trim_Verification/Missile_Plant_Trim/Missile Dynamics/Aerodynamic Forces and Moments/Compute Body Frame Aerodynamic Forces and Moments/Compute Aeroballistics Frame Aerodynamics Coefficients/Calculate Coefficient Parameters/Compose ROT_b_to_a ==
  roll_angle_T : Inport
  11 : Constant
  {12..13,21,31} (4 alike) : Constant  Value=0
  22 : Trigonometry  Operator=cos
  23 : Trigonometry
  32 : Trigonometry
  33 : Trigonometry  Operator=cos
  Create 3x3 Matrix : sharedutil/Create 3x3 Matrix  aMode=aMode
      settings: SourceProductBaseCode=AE,PW,DR,MT,UV,VE
  Gain : Gain  Gain=-1
  ROT_b_to_a : Outport
  wires:
  Create 3x3 Matrix/1 -> ROT_b_to_a/1
  33/1 -> Create 3x3 Matrix/9
  32/1 -> Create 3x3 Matrix/8
  31/1 -> Create 3x3 Matrix/7
  Gain/1 -> Create 3x3 Matrix/6
  22/1 -> Create 3x3 Matrix/5
  21/1 -> Create 3x3 Matrix/4
  13/1 -> Create 3x3 Matrix/3
  12/1 -> Create 3x3 Matrix/2
  11/1 -> Create 3x3 Matrix/1
  23/1 -> Gain/1
  roll_angle_T/1 -> 22/1, 23/1, 32/1, 33/1

== system Missile_Trim_Verification/Missile_Plant_Trim/Missile Dynamics/Aerodynamic Forces and Moments/Compute Body Frame Aerodynamic Forces and Moments/Compute Aeroballistics Frame Aerodynamics Coefficients/Calculate Coefficient Parameters/Convert CtrlSurfaces[b] to CtrlSurfaces[b][a] ==
  ROT_b_to_a : Inport
  CtrlSurfaces[b] : Inport  Port=2
  Matrix Multiply : Product  Multiplication=Matrix(*)
  CtrlSurfaces[a] : Outport
  wires:
  CtrlSurfaces[b]/1 -> Matrix Multiply/2
  ROT_b_to_a/1 -> Matrix Multiply/1
  Matrix Multiply/1 -> CtrlSurfaces[a]/1

== system Missile_Trim_Verification/Missile_Plant_Trim/Missile Dynamics/Aerodynamic Forces and Moments/Compute Body Frame Aerodynamic Forces and Moments/Compute Aeroballistics Frame Aerodynamics Coefficients/Calculate Coefficient Parameters/Convert pqr[b] to pqr[a] ==
  ROT_b_to_a : Inport
  pqr[b] : Inport  Port=2
  Matrix Multiply : Product  Multiplication=Matrix(*)
  pqr[a] : Outport
  wires:
  pqr[b]/1 -> Matrix Multiply/2
  ROT_b_to_a/1 -> Matrix Multiply/1
  Matrix Multiply/1 -> pqr[a]/1

== system Missile_Trim_Verification/Missile_Plant_Trim/Missile Dynamics/Aerodynamic Forces and Moments/Compute Body Frame Aerodynamic Forces and Moments/Compute Aeroballistics Frame Aerodynamics Coefficients/Calculate Coefficient Parameters/Subsystem ==
  D : Inport
  Divide : Product  Inputs=*/
  Minus : Sum  Inputs=+-
  Missile C.G. Point : Constant  Value=XCG
  Missile Moment Reference Point : Constant  Value=XREF
  geo_param : Outport
  wires:
  Minus/1 -> Divide/1
  Divide/1 -> geo_param/1
  D/1 -> Divide/2
  Missile Moment Reference Point/1 -> Minus/2
  Missile C.G. Point/1 -> Minus/1

== system Missile_Trim_Verification/Missile_Plant_Trim/Missile Dynamics/Aerodynamic Forces and Moments/Compute Body Frame Aerodynamic Forces and Moments/Compute Aeroballistics Frame Aerodynamics Coefficients/Compute Aero-F-Coeffs_a/Compute CX_a ==
  Mach_Number_index : Inport
  alpha_T : Inport  Port=2
  dEFF : Inport  Port=3
  Add : Sum  Inputs=+++
  Bus Selector : BusSelector  OutputSignals=k,f
  CX_0 : Interpolation_n-D  NumberOfTableDimensions=1  Table=Tbl_CX_0  InternalRulePriority=Speed
      settings: InputPortMap=u0,u1
  CX_ALPHAT : Interpolation_n-D  NumberOfTableDimensions=1  Table=Tbl_CX_ALPHAT  InternalRulePriority=Speed
      settings: InputPortMap=u0,u1
  CX_DEL_EFF : Interpolation_n-D  NumberOfTableDimensions=1  Table=Tbl_CX_DEL_EFF  InternalRulePriority=Speed
      settings: InputPortMap=u0,u1
  Math Function : Math  Operator=square  SaturateOnIntegerOverflow=on
  Product : Product
  Product1 : Product
  CX_a : Outport
  wires:
  Add/1 -> CX_a/1
  Product1/1 -> Add/3
  Product/1 -> Add/2
  CX_0/1 -> Add/1
  Math Function/1 -> Product1/2
  CX_DEL_EFF/1 -> Product1/1
  dEFF/1 -> Math Function/1
  alpha_T/1 -> Product/2
  CX_ALPHAT/1 -> Product/1
  Bus Selector/2 -> CX_0/2, CX_ALPHAT/2, CX_DEL_EFF/2  "<f>"
  Bus Selector/1 -> CX_0/1, CX_ALPHAT/1, CX_DEL_EFF/1  "<k>"
  Mach_Number_index/1 -> Bus Selector/1

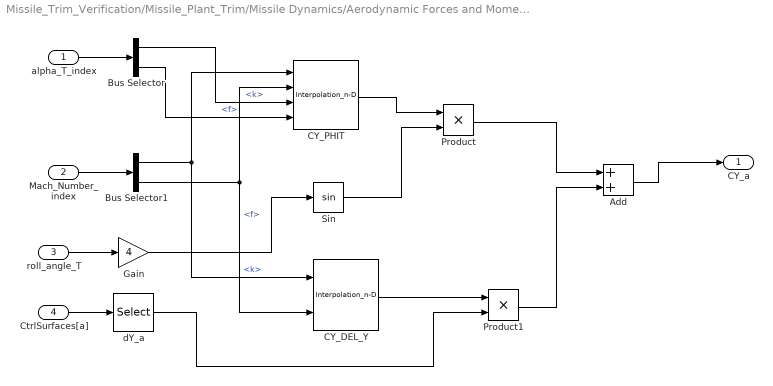
== system Missile_Trim_Verification/Missile_Plant_Trim/Missile Dynamics/Aerodynamic Forces and Moments/Compute Body Frame Aerodynamic Forces and Moments/Compute Aeroballistics Frame Aerodynamics Coefficients/Compute Aero-F-Coeffs_a/Compute CY_a ==
  alpha_T_index : Inport
  Mach_Number_index : Inport  Port=2
  roll_angle_T : Inport  Port=3
  CtrlSurfaces[a] : Inport  Port=4
  Add : Sum
  Bus Selector : BusSelector  OutputSignals=k,f
  Bus Selector1 : BusSelector  OutputSignals=k,f
  CY_DEL_Y : Interpolation_n-D  NumberOfTableDimensions=1  Table=Tbl_CY_DEL_Y  InternalRulePriority=Speed
      settings: InputPortMap=u0,u1
  CY_PHIT : Interpolation_n-D  Table=Tbl_CY_PHIT  InternalRulePriority=Speed
  Gain : Gain  Gain=4
  Product : Product
  Product1 : Product
  Sin : Trigonometry
  dY_a : Selector  InputPortWidth=3  IndexOptions=Index vector (dialog)  Indices=[3]  OutputSizes=1
  CY_a : Outport
  wires:
  Bus Selector/2 -> CY_PHIT/4  "<f>"
  Bus Selector/1 -> CY_PHIT/3  "<k>"
  Add/1 -> CY_a/1
  Product1/1 -> Add/2
  dY_a/1 -> Product1/2
  CY_DEL_Y/1 -> Product1/1
  Product/1 -> Add/1
  Sin/1 -> Product/2
  Gain/1 -> Sin/1
  roll_angle_T/1 -> Gain/1
  CY_PHIT/1 -> Product/1
  Bus Selector1/2 -> CY_DEL_Y/2, CY_PHIT/2  "<f>"
  Bus Selector1/1 -> CY_DEL_Y/1, CY_PHIT/1  "<k>"
  CtrlSurfaces[a]/1 -> dY_a/1
  Mach_Number_index/1 -> Bus Selector1/1
  alpha_T_index/1 -> Bus Selector/1

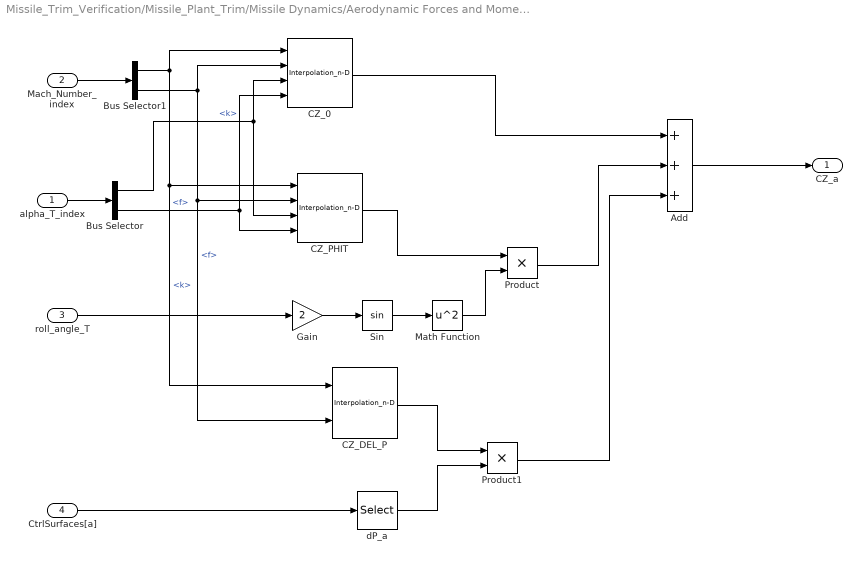
== system Missile_Trim_Verification/Missile_Plant_Trim/Missile Dynamics/Aerodynamic Forces and Moments/Compute Body Frame Aerodynamic Forces and Moments/Compute Aeroballistics Frame Aerodynamics Coefficients/Compute Aero-F-Coeffs_a/Compute CZ_a ==
  alpha_T_index : Inport
  Mach_Number_index : Inport  Port=2
  roll_angle_T : Inport  Port=3
  CtrlSurfaces[a] : Inport  Port=4
  Add : Sum  Inputs=+++
  Bus Selector : BusSelector  OutputSignals=k,f
  Bus Selector1 : BusSelector  OutputSignals=k,f
  CZ_0 : Interpolation_n-D  Table=Tbl_CZ_0  InternalRulePriority=Speed
  CZ_DEL_P : Interpolation_n-D  NumberOfTableDimensions=1  Table=Tbl_CZ_DEL_P  InternalRulePriority=Speed
      settings: InputPortMap=u0,u1
  CZ_PHIT : Interpolation_n-D  Table=Tbl_CZ_PHIT  InternalRulePriority=Speed
  Gain : Gain  Gain=2
  Math Function : Math  Operator=square  SaturateOnIntegerOverflow=on
  Product : Product
  Product1 : Product
  Sin : Trigonometry
  dP_a : Selector  InputPortWidth=3  IndexOptions=Index vector (dialog)  Indices=[2]  OutputSizes=1
  CZ_a : Outport
  wires:
  Bus Selector/2 -> CZ_0/4, CZ_PHIT/4  "<f>"
  Bus Selector/1 -> CZ_0/3, CZ_PHIT/3  "<k>"
  Add/1 -> CZ_a/1
  Product1/1 -> Add/3
  Product/1 -> Add/2
  CZ_0/1 -> Add/1
  dP_a/1 -> Product1/2
  CZ_DEL_P/1 -> Product1/1
  Math Function/1 -> Product/2
  CZ_PHIT/1 -> Product/1
  Sin/1 -> Math Function/1
  Gain/1 -> Sin/1
  roll_angle_T/1 -> Gain/1
  Bus Selector1/2 -> CZ_0/2, CZ_PHIT/2, CZ_DEL_P/2  "<f>"
  Bus Selector1/1 -> CZ_0/1, CZ_PHIT/1, CZ_DEL_P/1  "<k>"
  CtrlSurfaces[a]/1 -> dP_a/1
  Mach_Number_index/1 -> Bus Selector1/1
  alpha_T_index/1 -> Bus Selector/1

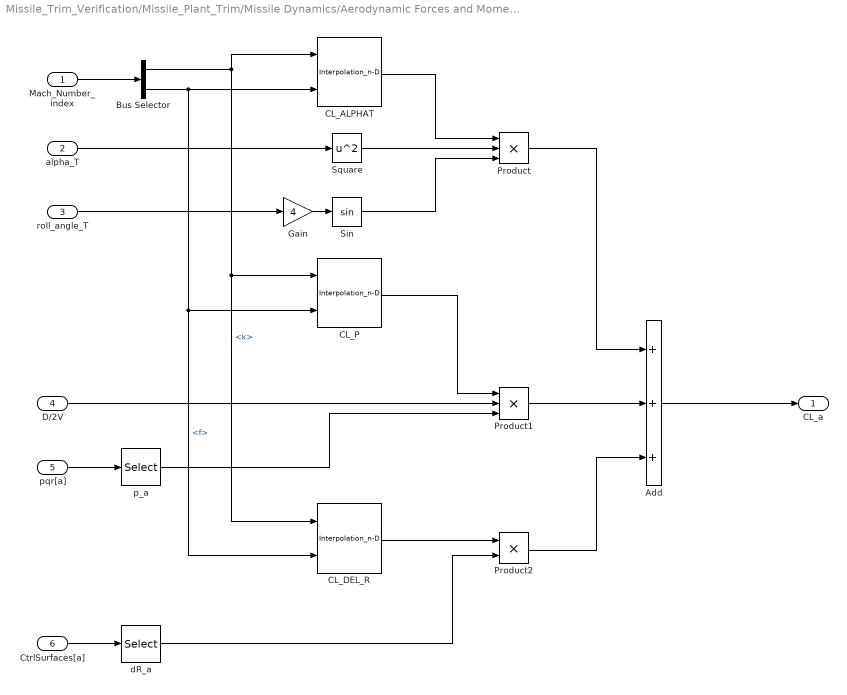
== system Missile_Trim_Verification/Missile_Plant_Trim/Missile Dynamics/Aerodynamic Forces and Moments/Compute Body Frame Aerodynamic Forces and Moments/Compute Aeroballistics Frame Aerodynamics Coefficients/Compute Aero-M-Coeffs_a/Compute CL_a ==
  Mach_Number_index : Inport
  alpha_T : Inport  Port=2
  roll_angle_T : Inport  Port=3
  D/2V : Inport  Port=4
  pqr[a] : Inport  Port=5
  CtrlSurfaces[a] : Inport  Port=6
  Add : Sum  Inputs=+++
  Bus Selector : BusSelector  OutputSignals=k,f
  CL_ALPHAT : Interpolation_n-D  NumberOfTableDimensions=1  Table=Tbl_CL_ALPHAT  InternalRulePriority=Speed
      settings: InputPortMap=u0,u1
  CL_DEL_R : Interpolation_n-D  NumberOfTableDimensions=1  Table=Tbl_CL_DEL_R  InternalRulePriority=Speed
      settings: InputPortMap=u0,u1
  CL_P : Interpolation_n-D  NumberOfTableDimensions=1  Table=Tbl_CL_P  InternalRulePriority=Speed
      settings: InputPortMap=u0,u1
  Gain : Gain  Gain=4
  Product : Product  Inputs=3
  Product1 : Product  Inputs=3
  Product2 : Product
  Sin : Trigonometry
  Square : Math  Operator=square  SaturateOnIntegerOverflow=on
  dR_a : Selector  InputPortWidth=3  IndexOptions=Index vector (dialog)  Indices=[1]  OutputSizes=1
  p_a : Selector  InputPortWidth=3  IndexOptions=Index vector (dialog)  Indices=[1]  OutputSizes=1
  CL_a : Outport
  wires:
  Add/1 -> CL_a/1
  Product2/1 -> Add/3
  Product1/1 -> Add/2
  Product/1 -> Add/1
  dR_a/1 -> Product2/2
  CL_DEL_R/1 -> Product2/1
  CtrlSurfaces[a]/1 -> dR_a/1
  p_a/1 -> Product1/3
  D/2V/1 -> Product1/2
  CL_P/1 -> Product1/1
  pqr[a]/1 -> p_a/1
  Sin/1 -> Product/3
  Square/1 -> Product/2
  CL_ALPHAT/1 -> Product/1
  Gain/1 -> Sin/1
  roll_angle_T/1 -> Gain/1
  alpha_T/1 -> Square/1
  Bus Selector/2 -> CL_ALPHAT/2, CL_P/2, CL_DEL_R/2  "<f>"
  Bus Selector/1 -> CL_ALPHAT/1, CL_P/1, CL_DEL_R/1  "<k>"
  Mach_Number_index/1 -> Bus Selector/1

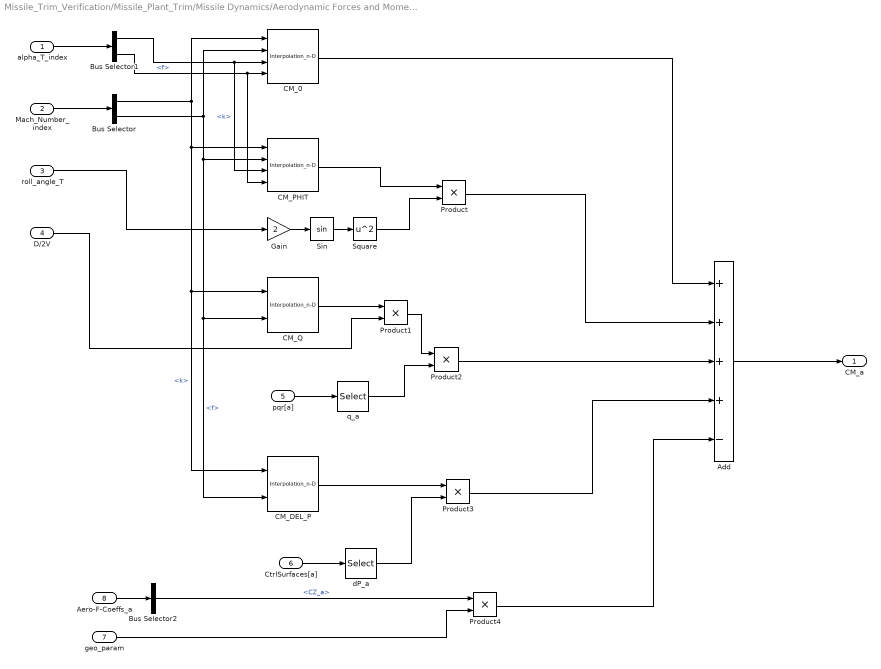
== system Missile_Trim_Verification/Missile_Plant_Trim/Missile Dynamics/Aerodynamic Forces and Moments/Compute Body Frame Aerodynamic Forces and Moments/Compute Aeroballistics Frame Aerodynamics Coefficients/Compute Aero-M-Coeffs_a/Compute CM_a ==
  alpha_T_index : Inport
  Mach_Number_index : Inport  Port=2
  roll_angle_T : Inport  Port=3
  D/2V : Inport  Port=4
  pqr[a] : Inport  Port=5
  CtrlSurfaces[a] : Inport  Port=6
  geo_param : Inport  Port=7
  Aero-F-Coeffs_a : Inport  Port=8
  Add : Sum  Inputs=++++-
  Bus Selector : BusSelector  OutputSignals=k,f
  Bus Selector1 : BusSelector  OutputSignals=k,f
  Bus Selector2 : BusSelector  OutputSignals=CZ_a
  CM_0 : Interpolation_n-D  Table=Tbl_CM_0  InternalRulePriority=Speed
  CM_DEL_P : Interpolation_n-D  NumberOfTableDimensions=1  Table=Tbl_CM_DEL_P  InternalRulePriority=Speed
      settings: InputPortMap=u0,u1
  CM_PHIT : Interpolation_n-D  Table=Tbl_CM_PHIT  InternalRulePriority=Speed
  CM_Q : Interpolation_n-D  NumberOfTableDimensions=1  Table=Tbl_CM_Q  InternalRulePriority=Speed
      settings: InputPortMap=u0,u1
  Gain : Gain  Gain=2
  Product{,1..4} (5 alike) : Product
  Sin : Trigonometry
  Square : Math  Operator=square  SaturateOnIntegerOverflow=on
  dP_a : Selector  InputPortWidth=3  IndexOptions=Index vector (dialog)  Indices=[2]  OutputSizes=1
  q_a : Selector  InputPortWidth=3  IndexOptions=Index vector (dialog)  Indices=[2]  OutputSizes=1
  CM_a : Outport
  wires:
  Bus Selector1/2 -> CM_PHIT/4, CM_0/4  "<f>"
  Bus Selector1/1 -> CM_PHIT/3, CM_0/3  "<k>"
  Add/1 -> CM_a/1
  Product4/1 -> Add/5
  Product3/1 -> Add/4
  Product2/1 -> Add/3
  Product/1 -> Add/2
  CM_0/1 -> Add/1
  geo_param/1 -> Product4/2
  Bus Selector2/1 -> Product4/1  "<CZ_a>"
  Aero-F-Coeffs_a/1 -> Bus Selector2/1
  dP_a/1 -> Product3/2
  CM_DEL_P/1 -> Product3/1
  q_a/1 -> Product2/2
  Product1/1 -> Product2/1
  D/2V/1 -> Product1/2
  CM_Q/1 -> Product1/1
  Square/1 -> Product/2
  CM_PHIT/1 -> Product/1
  Sin/1 -> Square/1
  Gain/1 -> Sin/1
  roll_angle_T/1 -> Gain/1
  Bus Selector/2 -> CM_0/2, CM_PHIT/2, CM_DEL_P/2, CM_Q/2  "<f>"
  Bus Selector/1 -> CM_0/1, CM_PHIT/1, CM_Q/1, CM_DEL_P/1  "<k>"
  alpha_T_index/1 -> Bus Selector1/1
  CtrlSurfaces[a]/1 -> dP_a/1
  pqr[a]/1 -> q_a/1
  Mach_Number_index/1 -> Bus Selector/1

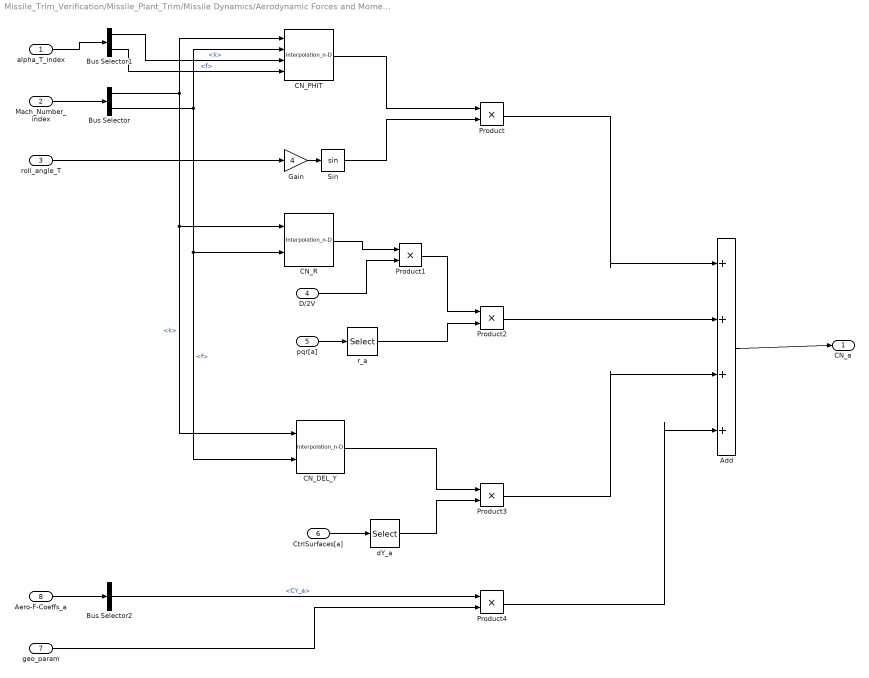
== system Missile_Trim_Verification/Missile_Plant_Trim/Missile Dynamics/Aerodynamic Forces and Moments/Compute Body Frame Aerodynamic Forces and Moments/Compute Aeroballistics Frame Aerodynamics Coefficients/Compute Aero-M-Coeffs_a/Compute CN_a ==
  alpha_T_index : Inport
  Mach_Number_index : Inport  Port=2
  roll_angle_T : Inport  Port=3
  D/2V : Inport  Port=4
  pqr[a] : Inport  Port=5
  CtrlSurfaces[a] : Inport  Port=6
  geo_param : Inport  Port=7
  Aero-F-Coeffs_a : Inport  Port=8
  Add : Sum  Inputs=++++
  Bus Selector : BusSelector  OutputSignals=k,f
  Bus Selector1 : BusSelector  OutputSignals=k,f
  Bus Selector2 : BusSelector  OutputSignals=CY_a
  CN_DEL_Y : Interpolation_n-D  NumberOfTableDimensions=1  Table=Tbl_CN_DEL_Y  InternalRulePriority=Speed
      settings: InputPortMap=u0,u1
  CN_PHIT : Interpolation_n-D  Table=Tbl_CN_PHIT  InternalRulePriority=Speed
  CN_R : Interpolation_n-D  NumberOfTableDimensions=1  Table=Tbl_CN_R  InternalRulePriority=Speed
      settings: InputPortMap=u0,u1
  Gain : Gain  Gain=4
  Product{,1..4} (5 alike) : Product
  Sin : Trigonometry
  dY_a : Selector  InputPortWidth=3  IndexOptions=Index vector (dialog)  Indices=[3]  OutputSizes=1
  r_a : Selector  InputPortWidth=3  IndexOptions=Index vector (dialog)  Indices=[3]  OutputSizes=1
  CN_a : Outport
  wires:
  Bus Selector1/2 -> CN_PHIT/4  "<f>"
  Bus Selector1/1 -> CN_PHIT/3  "<k>"
  Add/1 -> CN_a/1
  Product4/1 -> Add/4
  Product3/1 -> Add/3
  Product2/1 -> Add/2
  Product/1 -> Add/1
  geo_param/1 -> Product4/2
  Bus Selector2/1 -> Product4/1  "<CY_a>"
  dY_a/1 -> Product3/2
  CN_DEL_Y/1 -> Product3/1
  CtrlSurfaces[a]/1 -> dY_a/1
  r_a/1 -> Product2/2
  Product1/1 -> Product2/1
  pqr[a]/1 -> r_a/1
  D/2V/1 -> Product1/2
  CN_R/1 -> Product1/1
  Sin/1 -> Product/2
  CN_PHIT/1 -> Product/1
  Gain/1 -> Sin/1
  roll_angle_T/1 -> Gain/1
  Bus Selector/2 -> CN_DEL_Y/2, CN_R/2, CN_PHIT/2  "<f>"
  Bus Selector/1 -> CN_DEL_Y/1, CN_R/1, CN_PHIT/1  "<k>"
  Aero-F-Coeffs_a/1 -> Bus Selector2/1
  alpha_T_index/1 -> Bus Selector1/1
  Mach_Number_index/1 -> Bus Selector/1

== matlab function Missile_Trim_Verification/Missile_Plant_Trim/Missile Dynamics/Augmented States for Trim Analysis/Compute CTC ==
  data: u input; y output size=1
function y = fcn(u)

y = sin(u(4))-u(7)*cos(u(2))*(sin(u(1))*tan(u(5))+cos(u(1))*cos(u(4)));

== matlab function Missile_Trim_Verification/Missile_Plant_Trim/Missile Dynamics/Augmented States for Trim Analysis/Compute [b] ==
  data: u input; b output
function b = fcn(u)

b = sin(u(4))*sin(u(2))+cos(u(4))*sin(u(1))*cos(u(2));

== matlab function Missile_Trim_Verification/Missile_Plant_Trim/Missile Dynamics/Augmented States for Trim Analysis/Compute ROC ==
  data: u input; y output size=1
function y = fcn(u)

y = sin(u(4))-u(1)*sin(u(3))+u(2)*cos(u(3));

== matlab function Missile_Trim_Verification/Missile_Plant_Trim/Missile Dynamics/Augmented States for Trim Analysis/Compute [a] ==
  data: u input; a output
function a = fcn(u)

a = cos(u(1))*cos(u(2));
